simulink model "Copy_of_realtime"  (R2024b)
settings: Solver=ode5  StartTime=0.0  StopTime=10  FixedStep=0.001  RelTol=1e-3
values from neighbouring files (symbols this model uses):
  A = [0, 1; 0, -1/Tm]    [DesignPart567.m]    (also in DesignPart8.m; DesignPart9Sine.m; DesignPart9Step.m = [0, 1; 0, a22]; Init.m = [0, 1;0, -1/Tm])
  B = [0, km/(gbox.N*Tm)]'    [DesignPart567.m]    (also in DesignPart8.m; DesignPart9Sine.m; DesignPart9Step.m = [0, b2]'; Init.m = [0; drv.dcgain*mot.Kt/(gbox.N1*mot.Req*Jeq)])
  C = [1, 0]    [DesignPart567.m]    (also in DesignPart8.m; DesignPart9Sine.m; DesignPart9Step.m; Init.m)
  Cr = [90, 0]    [DesignPart567.m]    (also in DesignPart8.m = 90)
  delta_est = 1/sqrt(2)    [DesignPart9Step.m]    (also in Init.m)
  K = real(K)    [DesignPart567.m]    (also in DesignPart8.m; DesignPart9Sine.m; DesignPart9Step.m = place(  A,   B, CtrlPoles); Init.m = acker(A,B,poles))
  W0 = 1/Tr    (= 10)    [DesignPart567.m]    (also in DesignPart9Sine.m = 2*pi/Tr)
  wc = 2*pi*50    (= 314.159265359)    [DesignPart9Step.m]    (also in Init.m; State_space_1324.m)
undefined symbols (not defined in the file or in its folder): National_Instruments, PCI, sens
libraries: simulink_extras x3, sldrtlib x3
settings Model: SimulationMode=external  ExtModeTrigDuration=1000001  Creator=galeazzolu  LastModifiedBy=galeazzolu
settings DataIOCC: ReturnWorkspaceOutputs=off
settings HardwareCC: ProdBitPerLong=64  ProdHWDeviceType=Intel->x86-64 (Linux 64)
settings RTWCC: Description=Simulink Desktop Real-Time  SystemTargetFile=sldrt.tlc  TemplateMakefile=sldrt.tmf  RTWCompilerOptimization=on
settings CodeAppCC: MaxIdLength=95
settings SimulinkDesktopRealTimeCC: TargetLibSuffix=_sldrt.a  TargetPreCompLibLocation=C:\Program Files\MATLAB\R2024b\toolbox\sldrt\lib\win64  ParMdlRefBuildCompliant=on

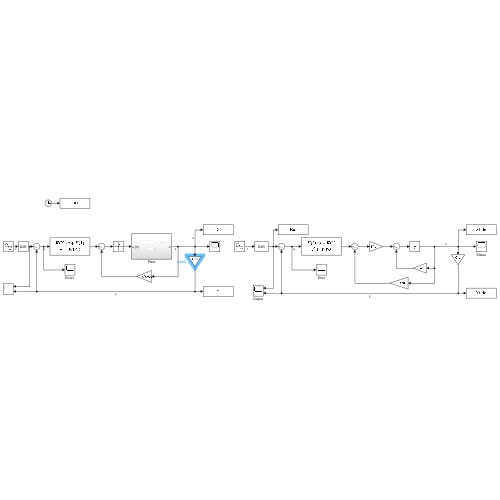
[thumbnail: Simulink's stored preview of the top-level diagram]
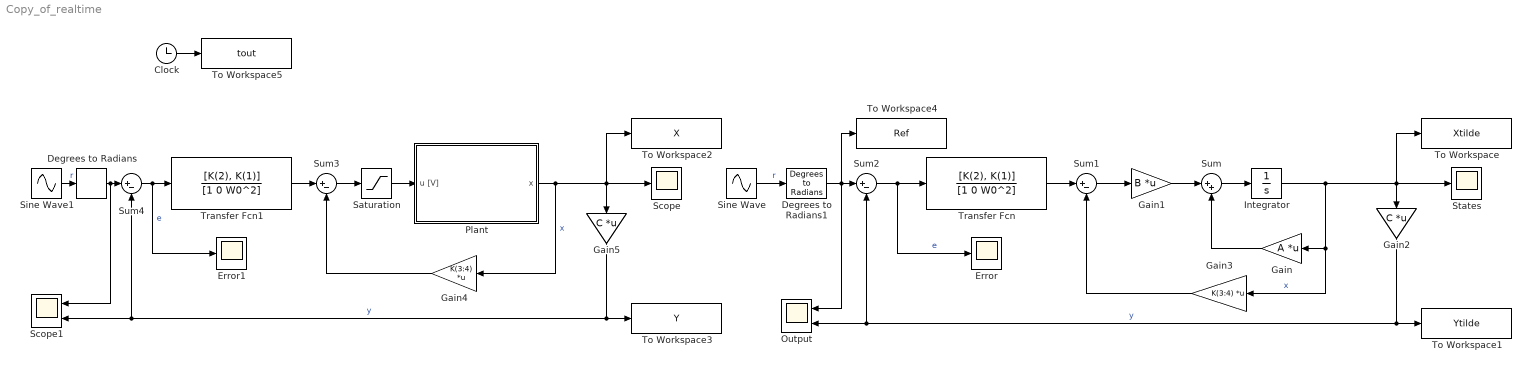
== system Copy_of_realtime ==
  Clock : Clock
  Degrees to Radians : simulink_extras/Transformations/Degrees to Radians
  Degrees to Radians1 : simulink_extras/Transformations/Degrees to Radians
  Error : Scope
  Error1 : Scope
  Gain : Gain  Gain=A  Multiplication=Matrix(K*u)
  Gain1 : Gain  Gain=B  Multiplication=Matrix(K*u)
  Gain2 : Gain  Gain=C  Multiplication=Matrix(K*u)
  Gain3 : Gain  Gain=K(3:4)  Multiplication=Matrix(K*u)
  Gain4 : Gain  Gain=K(3:4)  Multiplication=Matrix(K*u) (u vector)
  Gain5 : Gain  Gain=C  Multiplication=Matrix(K*u)
  Integrator : Integrator  InitialCondition=rand(2, 1)
  Output : Scope  NumInputPorts=2
  Plant : Subsystem
  Saturation : Saturate  UpperLimit=10  LowerLimit=-10
  Scope : Scope
  Scope1 : Scope  NumInputPorts=2
  Sine Wave : Sin  Amplitude=Cr(1)  Frequency=W0  SampleTime=0
  Sine Wave1 : Sin  Amplitude=Cr(1)  Frequency=W0  SampleTime=0
  States : Scope
  Sum : Sum  Inputs=|++
  Sum{1..4} (4 alike) : Sum  Inputs=|+-
  To Workspace : ToWorkspace  VariableName=Xtilde  SaveFormat=Timeseries  SampleTime=-1
  To Workspace1 : ToWorkspace  VariableName=Ytilde  SaveFormat=Timeseries  SampleTime=-1
  To Workspace2 : ToWorkspace  VariableName=X  SaveFormat=Timeseries  SampleTime=-1
  To Workspace3 : ToWorkspace  VariableName=Y  SaveFormat=Timeseries  SampleTime=-1
  To Workspace4 : ToWorkspace  VariableName=Ref  SaveFormat=Timeseries  SampleTime=-1
  To Workspace5 : ToWorkspace  VariableName=tout  SaveFormat=Timeseries  SampleTime=-1
  Transfer Fcn : TransferFcn  Numerator=[K(2), K(1)]  Denominator=[1 0 W0^2]
  Transfer Fcn1 : TransferFcn  Numerator=[K(2), K(1)]  Denominator=[1 0 W0^2]
  wires:
  Transfer Fcn1/1 -> Sum3/1
  Sine Wave1/1 -> Degrees to Radians/1  "r"
  Gain/1 -> Sum/2
  Sum3/1 -> Saturation/1
  Plant/1(x) -> To Workspace2/1, Gain5/1, Scope/1, Gain4/1  "x"
  Sum2/1 -> Error/1, Transfer Fcn/1  "e"
  Gain1/1 -> Sum/1
  Sum/1 -> Integrator/1
  Sine Wave/1 -> Degrees to Radians1/1  "r"
  Integrator/1 -> Gain/1, Gain3/1, To Workspace/1, Gain2/1, States/1  "x"
  Degrees to Radians1/1 -> Output/1, To Workspace4/1, Sum2/1
  Degrees to Radians/1 -> Scope1/1, Sum4/1
  Sum4/1 -> Transfer Fcn1/1, Error1/1  "e"
  Gain5/1 -> To Workspace3/1, Scope1/2, Sum4/2  "y"
  Sum1/1 -> Gain1/1
  Saturation/1 -> Plant/1(u [V])
  Gain4/1 -> Sum3/2
  Gain2/1 -> To Workspace1/1, Sum2/2, Output/2  "y"
  Gain3/1 -> Sum1/2
  Transfer Fcn/1 -> Sum1/1
  Clock/1 -> To Workspace5/1

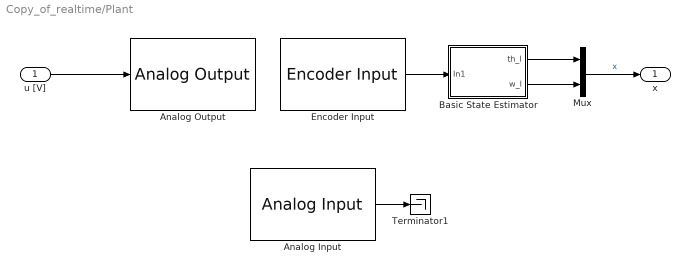
== system Copy_of_realtime/Plant ==
  u [V] : Inport
  Analog Input : sldrtlib/Analog Input  SampleTime=-1  MaxMissedTicks=10  ShowMissedTicks=off  YieldWhenWaiting=off  DrvName=National_Instruments/PCI-6221  DrvAddress=4294967295  DrvOptions=[0 0 0 2 0]  Channels=[1,2]  RangeMode=1  VoltRange=1  DataType=1
      settings: AttributesFormatString=National Instruments\nPCI-6221 [auto]
  Analog Output : sldrtlib/Analog Output  SampleTime=-1  MaxMissedTicks=10  ShowMissedTicks=off  YieldWhenWaiting=off  DrvName=National_Instruments/PCI-6221  DrvAddress=4294967295  DrvOptions=[0 0 0 2 0]  Channels=1  RangeMode=1  VoltRange=1  InitialValue=0  FinalValue=0
      settings: AttributesFormatString=National Instruments\nPCI-6221 [auto]
  Basic State Estimator : Subsystem
  Encoder Input : sldrtlib/Encoder Input  SampleTime=-1  MaxMissedTicks=10  ShowMissedTicks=off  YieldWhenWaiting=off  DrvName=National_Instruments/PCI-6221  DrvAddress=4294967295  DrvOptions=[0 0 0 2 0]  Channels=1  QuadMode=3  IndexPulse=1  InputFilter=Inf  DataType=1
      settings: AttributesFormatString=National Instruments\nPCI-6221 [auto]
  Mux : Mux  Inputs=2
  Terminator1 : Terminator
  x : Outport
  wires:
  u [V]/1 -> Analog Output/1
  Encoder Input/1 -> Basic State Estimator/1(In1)
  Mux/1 -> x/1  "x"
  Basic State Estimator/1(th_l) -> Mux/1
  Basic State Estimator/2(w_l) -> Mux/2
  Analog Input/1 -> Terminator1/1

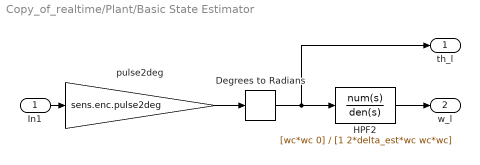
== system Copy_of_realtime/Plant/Basic State Estimator ==
  In1 : Inport
  Degrees to Radians : simulink_extras/Transformations/Degrees to Radians
  HPF2 : TransferFcn  Numerator=[wc*wc 0]  Denominator=[1 2*delta_est*wc wc*wc]
  pulse2deg : Gain  Gain=sens.enc.pulse2deg
  th_l : Outport
  w_l : Outport  Port=2
  wires:
  pulse2deg/1 -> Degrees to Radians/1
  In1/1 -> pulse2deg/1
  HPF2/1 -> w_l/1
  Degrees to Radians/1 -> th_l/1, HPF2/1
